simulink model "ARDSimpleModel"  (R2016a)
settings: Solver=ode3  StartTime=0.0  StopTime=0.1  FixedStep=0.1  RelTol=1e-3
undefined symbols (not defined in the file or in its folder): Euler2Quat, veh_prms
settings Model: SimulationMode=accelerator  Creator=ddiel  LastModifiedBy=ddiel
settings DataIOCC: ExternalInput=[x0; u]  FinalStateName=y  SaveFormat=Structure  SaveOutput=off  SignalLogging=off  DSMLogging=off  SaveTime=off  OutputSaveName=y
settings OptimizationCC: DefaultParameterBehavior=Inlined  SimCompilerOptimization=on
settings DebuggingCC: UnderspecifiedInitializationDetection=Classic  MergeDetectMultiDrivingBlocksExec=none  SolverPrmCheckMsg=warning
settings HardwareCC: ProdBitPerPointer=32  ProdLargestAtomicFloat=None  ProdIntDivRoundTo=Undefined  ProdEndianess=Unspecified  ProdWordSize=32  ProdHWDeviceType=32-bit Generic
settings ModelReferenceCC: PropagateSignalLabelsOutOfModel=off
settings ConfigComp: CovModelRefEnable=Off

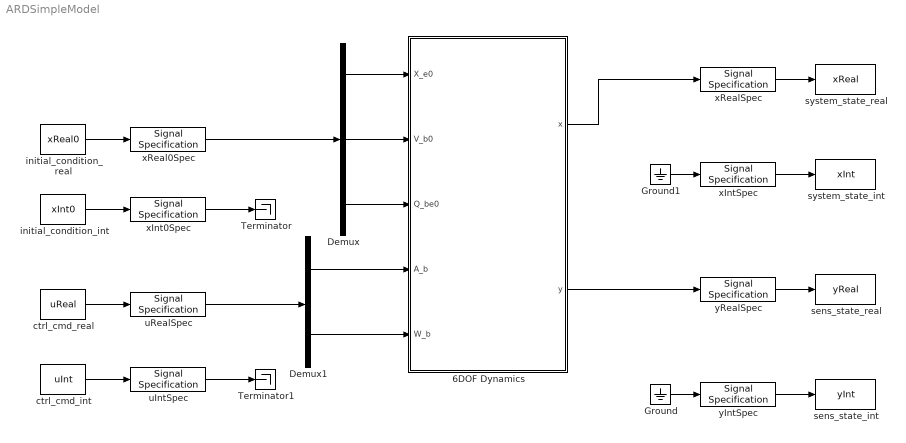
== system ARDSimpleModel ==
  6DOF Dynamics : Subsystem
  Demux : Demux  Outputs=[3,3,4]
  Demux1 : Demux  Outputs=[3,3]
  Ground : Ground
  Ground1 : Ground
  Terminator : Terminator
  Terminator1 : Terminator
  ctrl_cmd_int : FromWorkspace  VariableName=uInt  OutDataTypeStr=uint8  SampleTime=0.1  Interpolate=off  OutputAfterFinalValue=Holding final value
  ctrl_cmd_real : FromWorkspace  VariableName=uReal  OutDataTypeStr=double  SampleTime=0.1  Interpolate=off  OutputAfterFinalValue=Holding final value
  initial_condition_int : FromWorkspace  VariableName=xInt0  OutDataTypeStr=uint8  SampleTime=0.1  Interpolate=off  OutputAfterFinalValue=Holding final value
  initial_condition_real : FromWorkspace  VariableName=xReal0  OutDataTypeStr=double  SampleTime=0.1  Interpolate=off  OutputAfterFinalValue=Holding final value
  sens_state_int : ToWorkspace  VariableName=yInt  SampleTime=-1
      settings: MaxDataPoints=1
  sens_state_real : ToWorkspace  VariableName=yReal  SampleTime=-1
      settings: MaxDataPoints=1
  system_state_int : ToWorkspace  VariableName=xInt  SampleTime=-1
      settings: MaxDataPoints=1
  system_state_real : ToWorkspace  VariableName=xReal  SampleTime=-1
      settings: MaxDataPoints=1
  uIntSpec : SignalSpecification  OutDataTypeStr=uint8  Dimensions=1
  uRealSpec : SignalSpecification  OutDataTypeStr=double  Dimensions=6
  xInt0Spec : SignalSpecification  OutDataTypeStr=uint8  Dimensions=1
  xIntSpec : SignalSpecification  OutDataTypeStr=uint8  Dimensions=1
  xReal0Spec : SignalSpecification  OutDataTypeStr=double  Dimensions=10
  xRealSpec : SignalSpecification  OutDataTypeStr=double  Dimensions=10
  yIntSpec : SignalSpecification  OutDataTypeStr=uint8  Dimensions=1
  yRealSpec : SignalSpecification  OutDataTypeStr=double  Dimensions=15
  wires:
  Demux1/2 -> 6DOF Dynamics/5(W_b)
  Demux1/1 -> 6DOF Dynamics/4(A_b)
  Demux/1 -> 6DOF Dynamics/1(X_e0)
  Demux/3 -> 6DOF Dynamics/3(Q_be0)
  Demux/2 -> 6DOF Dynamics/2(V_b0)
  ctrl_cmd_real/1 -> uRealSpec/1
  initial_condition_real/1 -> xReal0Spec/1
  initial_condition_int/1 -> xInt0Spec/1
  ctrl_cmd_int/1 -> uIntSpec/1
  6DOF Dynamics/1(x) -> xRealSpec/1
  6DOF Dynamics/2(y) -> yRealSpec/1
  Ground/1 -> yIntSpec/1
  Ground1/1 -> xIntSpec/1
  xReal0Spec/1 -> Demux/1
  xInt0Spec/1 -> Terminator/1
  uRealSpec/1 -> Demux1/1
  uIntSpec/1 -> Terminator1/1
  xIntSpec/1 -> system_state_int/1
  xRealSpec/1 -> system_state_real/1
  yRealSpec/1 -> sens_state_real/1
  yIntSpec/1 -> sens_state_int/1

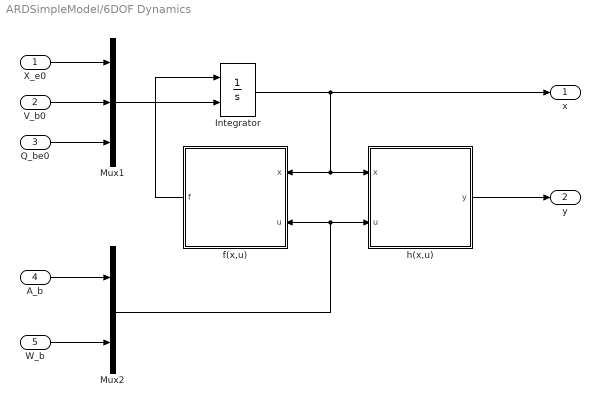
== system ARDSimpleModel/6DOF Dynamics ==
  X_e0 : Inport
  V_b0 : Inport  Port=2
  Q_be0 : Inport  Port=3
  A_b : Inport  Port=4
  W_b : Inport  Port=5
  Integrator : Integrator  InitialConditionSource=external  InitialCondition=[veh_prms.xo(1:6);Euler2Quat(veh_prms.xo(7:9))]  ContinuousStateAttributes='ARDSimpleModelIntegratorState'
  Mux1 : Mux  Inputs=[3, 3, 4]
  Mux2 : Mux  Inputs=[3, 3]
  f(x,u) : Subsystem
  h(x,u) : Subsystem
  x : Outport
  y : Outport  Port=2
  wires:
  A_b/1 -> Mux2/1
  W_b/1 -> Mux2/2
  Integrator/1 -> x/1, f(x,u)/1(x), h(x,u)/1(x)
  Mux2/1 -> f(x,u)/2(u), h(x,u)/2(u)
  h(x,u)/1(y) -> y/1
  f(x,u)/1(f) -> Integrator/1
  Mux1/1 -> Integrator/2
  X_e0/1 -> Mux1/1
  V_b0/1 -> Mux1/2
  Q_be0/1 -> Mux1/3

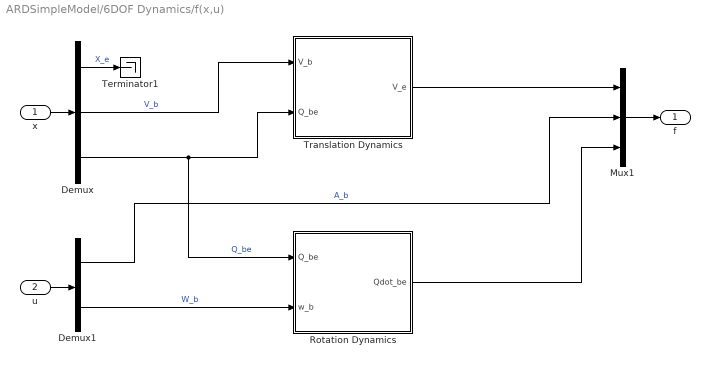
== system ARDSimpleModel/6DOF Dynamics/f(x,u) ==
  x : Inport
  u : Inport  Port=2
  Demux : Demux  Outputs=[3,3,4]
  Demux1 : Demux  Outputs=[3,3]
  Mux1 : Mux  Inputs=3
  Rotation Dynamics : Subsystem
  Terminator1 : Terminator
  Translation Dynamics : Subsystem
  f : Outport
  wires:
  Mux1/1 -> f/1
  Translation Dynamics/1(V_e) -> Mux1/1
  Rotation Dynamics/1(Qdot_be) -> Mux1/3
  x/1 -> Demux/1
  u/1 -> Demux1/1
  Demux/2 -> Translation Dynamics/1(V_b)  "V_b"
  Demux/3 -> Translation Dynamics/2(Q_be), Rotation Dynamics/1(Q_be)  "Q_be"
  Demux1/1 -> Mux1/2  "A_b"
  Demux1/2 -> Rotation Dynamics/2(w_b)  "W_b"
  Demux/1 -> Terminator1/1  "X_e"

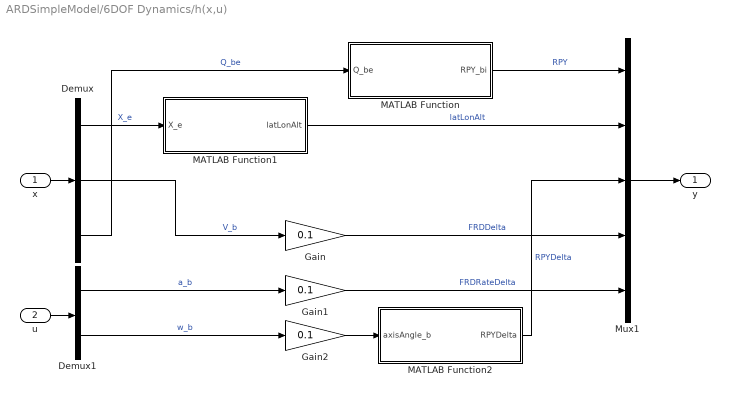
== system ARDSimpleModel/6DOF Dynamics/h(x,u) ==
  x : Inport
  u : Inport  Port=2
  Demux : Demux  Outputs=[3,3,4]
  Demux1 : Demux  Outputs=[3,3]
  Gain : Gain  Gain=0.1
  Gain1 : Gain  Gain=0.1
  Gain2 : Gain  Gain=0.1
  MATLAB Function : MATLAB Function  TreatAsAtomicUnit=on
  MATLAB Function1 : MATLAB Function  TreatAsAtomicUnit=on
  MATLAB Function2 : MATLAB Function  TreatAsAtomicUnit=on
  Mux1 : Mux  Inputs=5
  y : Outport
  wires:
  x/1 -> Demux/1
  Mux1/1 -> y/1
  Demux/3 -> MATLAB Function/1(Q_be)  "Q_be"
  u/1 -> Demux1/1
  MATLAB Function/1(RPY_bi) -> Mux1/1  "RPY"
  Demux/1 -> MATLAB Function1/1(X_e)  "X_e"
  MATLAB Function1/1(latLonAlt) -> Mux1/2  "latLonAlt"
  Demux/2 -> Gain/1  "V_b"
  Demux1/1 -> Gain1/1  "a_b"
  Demux1/2 -> Gain2/1  "w_b"
  Gain/1 -> Mux1/4  "FRDDelta"
  Gain1/1 -> Mux1/5  "FRDRateDelta"
  MATLAB Function2/1(RPYDelta) -> Mux1/3  "RPYDelta"
  Gain2/1 -> MATLAB Function2/1(axisAngle_b)

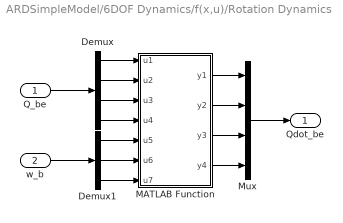
== system ARDSimpleModel/6DOF Dynamics/f(x,u)/Rotation Dynamics ==
  Q_be : Inport
  w_b : Inport  Port=2
  Demux : Demux
  Demux1 : Demux  Outputs=3
  MATLAB Function : MATLAB Function  TreatAsAtomicUnit=on
  Mux : Mux
  Qdot_be : Outport  PortDimensions=4
  wires:
  Demux/4 -> MATLAB Function/4(u4)
  Demux/1 -> MATLAB Function/1(u1)
  Demux/2 -> MATLAB Function/2(u2)
  Demux/3 -> MATLAB Function/3(u3)
  Q_be/1 -> Demux/1
  Demux1/1 -> MATLAB Function/5(u5)
  Demux1/2 -> MATLAB Function/6(u6)
  Demux1/3 -> MATLAB Function/7(u7)
  w_b/1 -> Demux1/1
  MATLAB Function/1(y1) -> Mux/1
  MATLAB Function/2(y2) -> Mux/2
  MATLAB Function/3(y3) -> Mux/3
  MATLAB Function/4(y4) -> Mux/4
  Mux/1 -> Qdot_be/1

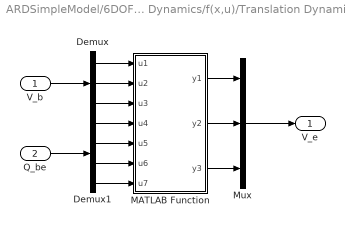
== system ARDSimpleModel/6DOF Dynamics/f(x,u)/Translation Dynamics ==
  V_b : Inport
  Q_be : Inport  Port=2
  Demux : Demux  Outputs=3
  Demux1 : Demux
  MATLAB Function : MATLAB Function  TreatAsAtomicUnit=on
  Mux : Mux  Inputs=3
  V_e : Outport  PortDimensions=3
  wires:
  V_b/1 -> Demux/1
  Demux/1 -> MATLAB Function/1(u1)
  Demux/2 -> MATLAB Function/2(u2)
  Demux/3 -> MATLAB Function/3(u3)
  Demux1/4 -> MATLAB Function/7(u7)
  Demux1/1 -> MATLAB Function/4(u4)
  Demux1/2 -> MATLAB Function/5(u5)
  Demux1/3 -> MATLAB Function/6(u6)
  Q_be/1 -> Demux1/1
  MATLAB Function/1(y1) -> Mux/1
  MATLAB Function/2(y2) -> Mux/2
  MATLAB Function/3(y3) -> Mux/3
  Mux/1 -> V_e/1

== matlab function ARDSimpleModel/6DOF Dynamics/f(x,u)/Translation Dynamics/MATLAB Function ==
  data: u1 input; y1 output; u2 input; u3 input; u4 input; u5 input; u6 input; u7 input; y2 output; y3 output
function [y1, y2, y3] = fcn(u1, u2, u3, u4, u5, u6, u7)
%#codegen
x = quatToMatrix(u4, u5, u6, u7)*[u1; u2; u3];
y1 = x(1);
y2 = x(2);
y3 = x(3);
end

function [qNorm0, qNorm1, qNorm2, qNorm3] = quatNorm(q0, q1, q2, q3)
qNorm0 = q0;
qNorm1 = q1;
qNorm2 = q2;
qNorm3 = q3;
n = sqrt(q0.*q0+q1.*q1+q2.*q2+q3.*q3);
small = find(n<eps);
qNorm0(small) = 1.0;
qNorm1(small) = 0.0;
qNorm2(small) = 0.0;
qNorm3(small) = 0.0;
n(small) = 1.0;
neg = find(qNorm0<0.0);
n(neg) = -n(neg);
qNorm0 = qNorm0./n;
qNorm1 = qNorm1./n;
qNorm2 = qNorm2./n;
qNorm3 = qNorm3./n;
end

function R = quatToMatrix(q0, q1, q2, q3)
[q0, q1, q2, q3] = quatNorm(q0, q1, q2, q3);
q00 = q0.*q0;
q11 = q1.*q1;
q22 = q2.*q2;
q33 = q3.*q3;
q01 = q0.*q1;
q12 = q1.*q2;
q23 = q2.*q3;
q03 = q0.*q3;
q02 = q0.*q2;
q13 = q1.*q3;
r00 = q00+q11-q22-q33;
r10 = 2.0*(q12+q03);
r20 = 2.0*(q13-q02);
r01 = 2.0*(q12-q03);
r11 = q00-q11+q22-q33;
r21 = 2.0*(q23+q01);
r02 = 2.0*(q13+q02);
r12 = 2.0*(q23-q01);
r22 = q00-q11-q22+q33;
R = [r00, r01, r02; r10, r11, r12; r20, r21, r22];
end

== matlab function ARDSimpleModel/6DOF Dynamics/f(x,u)/Rotation Dynamics/MATLAB Function ==
  data: u1 input; y1 output; u2 input; u3 input; u4 input; u5 input; u6 input; u7 input; y2 output; y3 output; y4 output
function [y1, y2, y3, y4] = fcn(u1, u2, u3, u4, u5, u6, u7)
%#codegen
wb = [u5; u6; u7];
ww = quatToMatrix(u1, u2, u3, u4)*wb;
x = 0.5*quatToHomo(u1, u2, u3, u4)*[0; ww];
y1 = x(1);
y2 = x(2);
y3 = x(3);
y4 = x(4);
end

function R = quatToMatrix(q0, q1, q2, q3)
[q0, q1, q2, q3] = quatNorm(q0, q1, q2, q3);
q00 = q0.*q0;
q11 = q1.*q1;
q22 = q2.*q2;
q33 = q3.*q3;
q01 = q0.*q1;
q12 = q1.*q2;
q23 = q2.*q3;
q03 = q0.*q3;
q02 = q0.*q2;
q13 = q1.*q3;
r00 = q00+q11-q22-q33;
r10 = 2.0*(q12+q03);
r20 = 2.0*(q13-q02);
r01 = 2.0*(q12-q03);
r11 = q00-q11+q22-q33;
r21 = 2.0*(q23+q01);
r02 = 2.0*(q13+q02);
r12 = 2.0*(q23-q01);
r22 = q00-q11-q22+q33;
R = [r00, r01, r02; r10, r11, r12; r20, r21, r22];
end

function [qNorm0, qNorm1, qNorm2, qNorm3] = quatNorm(q0, q1, q2, q3)
qNorm0 = q0;
qNorm1 = q1;
qNorm2 = q2;
qNorm3 = q3;
n = sqrt(q0.*q0+q1.*q1+q2.*q2+q3.*q3);
small = find(n<eps);
qNorm0(small) = 1.0;
qNorm1(small) = 0.0;
qNorm2(small) = 0.0;
qNorm3(small) = 0.0;
n(small) = 1.0;
neg = find(qNorm0<0.0);
n(neg) = -n(neg);
qNorm0 = qNorm0./n;
qNorm1 = qNorm1./n;
qNorm2 = qNorm2./n;
qNorm3 = qNorm3./n;
end

function h = quatToHomo(q0, q1, q2, q3)
[q0, q1, q2, q3] = quatNorm(q0, q1, q2, q3);
h = zeros(4, 4);
h(1, 1) = q0;
h(2, 1) = q1;
h(3, 1) = q2;
h(4, 1) = q3;
h(1, 2) = -q1;
h(2, 2) = q0;
h(3, 2) = q3;
h(4, 2) = -q2;
h(1, 3) = -q2;
h(2, 3) = -q3;
h(3, 3) = q0;
h(4, 3) = q1;
h(1, 4) = -q3;
h(2, 4) = q2;
h(3, 4) = -q1;
h(4, 4) = q0;
end

== matlab function ARDSimpleModel/6DOF Dynamics/h(x,u)/MATLAB Function ==
  data: Q_be input; RPY_bi output
function RPY_bi = fcn(Q_be)
%#codegen
betobi = quatToHomo(sqrt(2)/2, 0, sqrt(2)/2, 0);
Q_bi = betobi*[Q_be(1); Q_be(2); Q_be(3); Q_be(4)];
RPY_bi = quatToEuler(Q_bi)';
end   

function y = quatToEuler(q)
y = zeros(3, 1);
q0 = q(1);
q1 = q(2);
q2 = q(3);
q3 = q(4);
q00 = q0.*q0;
q11 = q1.*q1;
q22 = q2.*q2;
q33 = q3.*q3;
q01 = q0.*q1;
q12 = q1.*q2;
q23 = q2.*q3;
q03 = q0.*q3;
q02 = q0.*q2;
q13 = q1.*q3;
y(1) = atan2(2.0*(q23+q01), q00-q11-q22+q33);
y(2) = asin(min(max(-2.0*(q13-q02), -1.0), 1.0));
y(3) = atan2(2.0*(q12+q03), q00+q11-q22-q33);
end

function h = quatToHomo(q0, q1, q2, q3)
h = zeros(4, 4);
h(1, 1) = q0;
h(2, 1) = q1;
h(3, 1) = q2;
h(4, 1) = q3;
h(1, 2) = -q1;
h(2, 2) = q0;
h(3, 2) = q3;
h(4, 2) = -q2;
h(1, 3) = -q2;
h(2, 3) = -q3;
h(3, 3) = q0;
h(4, 3) = q1;
h(1, 4) = -q3;
h(2, 4) = q2;
h(3, 4) = -q1;
h(4, 4) = q0;
end

== matlab function ARDSimpleModel/6DOF Dynamics/h(x,u)/MATLAB Function1 ==
  data: X_e input; latLonAlt output
function latLonAlt = fcn(X_e)
%#codegen
x = X_e(1);
y = X_e(2);
z = X_e(3);
a = earth.WGS84.majorRadius;
finv = earth.WGS84.inverseFlattening;
f = 1.0/finv;
b = a-a/finv;
e2 = 2.0*f-f*f;
ep2 = f*(2.0-f)/((1.0-f)*(1.0-f));
r2 = x.*x+y.*y;
r = sqrt(r2);
E2 = a*a-b*b;
F = 54.0*b*b*z.*z;
G = r2+(1.0-e2)*z.*z-e2*E2;
c = (e2*e2*F.*r2)./(G.*G.*G);
s = power(1.0+c+sqrt(max(c.*c+2.0*c, 0.0)), 1.0/3.0);
P = F./(3.0*power(s+1./s+1, 2.0).*G.*G);
Q = sqrt(1.0+2.0*e2*e2*P);
ro = -(e2*P.*r)./(1.0+Q)+sqrt((a*a/2.0)*(1.0+1.0./Q)-((1.0-e2)*P.*z.*z)./(Q.*(1.0+Q))-P.*r2/2.0);
tmp = power(r-e2*ro, 2.0);
U = sqrt(tmp+z.*z);
V = sqrt(tmp+(1.0-e2)*z.*z);
zo = (b*b*z)./(a*V);
lon = atan2(y, x);
lat = atan2(z+ep2*zo, r);
alt = U.*(1.0-b*b./(a*V));
latLonAlt = [lat, lon, alt];
end

== matlab function ARDSimpleModel/6DOF Dynamics/h(x,u)/MATLAB Function2 ==
  data: axisAngle_b input; RPYDelta output
function RPYDelta = fcn(axisAngle_b)
%#codegen
aa = [axisAngle_b(1); axisAngle_b(2); axisAngle_b(3)];
aaNorm = sqrt(aa'*aa);
if(aaNorm<eps)
  quatDelta = [1; 0; 0; 0];
else
  halfAngle = aaNorm/2.0;
  quatDelta = [cos(halfAngle); aa/aaNorm*sin(halfAngle)];
end
RPYDelta = quatToEuler(quatDelta)';
end

function y = quatToEuler(q)
y = zeros(3, 1);
q0 = q(1);
q1 = q(2);
q2 = q(3);
q3 = q(4);
q00 = q0.*q0;
q11 = q1.*q1;
q22 = q2.*q2;
q33 = q3.*q3;
q01 = q0.*q1;
q12 = q1.*q2;
q23 = q2.*q3;
q03 = q0.*q3;
q02 = q0.*q2;
q13 = q1.*q3;
y(1) = atan2(2.0*(q23+q01), q00-q11-q22+q33);
y(2) = asin(min(max(-2.0*(q13-q02), -1.0), 1.0));
y(3) = atan2(2.0*(q12+q03), q00+q11-q22-q33);
end
